simulink model "check_serial_new_arduino_basic"  (R2021a)
settings: Solver=FixedStepDiscrete  StartTime=0.0  StopTime=inf  FixedStep=time_step  RelTol=1e-3
model workspace (MAT data in the model file):
  time_step = 0.01
undefined symbols (not defined in the file): Serial_Port, Standard_Devices
libraries: sldrtlib x2
settings Model: Creator=Rahul Subramanian  LastModifiedBy=Rahul Subramanian
settings SolverCC: AlgebraicLoopSolver=TrustRegion
settings DebuggingCC: SFMachineParentedDataDiag=warning
settings RTWCC: Description=Simulink Desktop Real-Time  SystemTargetFile=sldrt.tlc  TemplateMakefile=sldrt.tmf  RTWCompilerOptimization=on
settings CodeAppCC: MaxIdLength=95
settings SimulinkDesktopRealTimeCC: TargetPreCompLibLocation=C:\Program Files\MATLAB\R2021a\toolbox\sldrt\lib\win64

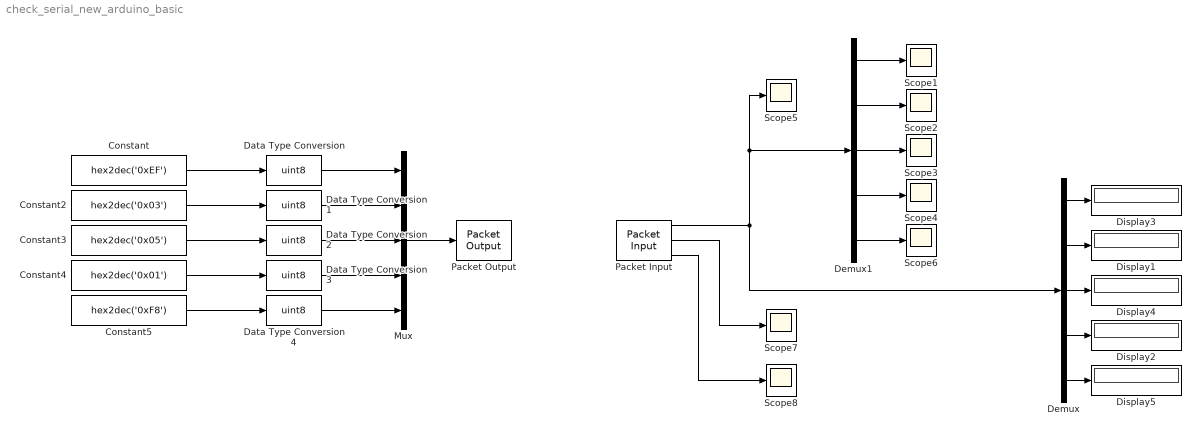
== system check_serial_new_arduino_basic ==
  Constant : Constant  Value=hex2dec('0xEF')
  Constant2 : Constant  Value=hex2dec('0x03')
  Constant3 : Constant  Value=hex2dec('0x05')
  Constant4 : Constant  Value=hex2dec('0x01')
  Constant5 : Constant  Value=hex2dec('0xF8')
  Data Type Conversion{,1..4} (5 alike) : DataTypeConversion  OutDataTypeStr=uint8
  Demux : Demux  Outputs=5
  Demux1 : Demux  Outputs=5
  Display{1..5} (5 alike) : Display
      settings: Format=hex (Stored Integer)
  Mux : Mux  Inputs=5
  Packet Input : sldrtlib/Packet Input  SampleTime=0.1  MaxMissedTicks=10  ShowMissedTicks=off  YieldWhenWaiting=off  DrvName=Standard_Devices/Serial_Port  DrvAddress=5  DrvOptions=[115200 8 0 0 0 0 0 0]  PacketSize=5  DataTypes='5*uint8'  ShowReady=on  ShowError=on  PacketID=1  ByteOrder=1  ShowTimestamp=off
      settings: AttributesFormatString=Serial Port [5]
  Packet Output : sldrtlib/Packet Output  SampleTime=0.1  MaxMissedTicks=10  ShowMissedTicks=off  YieldWhenWaiting=off  DrvName=Standard_Devices/Serial_Port  DrvAddress=5  DrvOptions=[115200 8 0 0 0 0 0 0]  PacketSize=5  DataTypes='5*uint8'  ShowReady=off  ShowError=off  PacketID=1  ByteOrder=1  InitialValue=[]  FinalValue=[]
      settings: AttributesFormatString=Serial Port [5]
  Scope{1..8} (8 alike) : Scope
  wires:
  Constant/1 -> Data Type Conversion/1
  Constant2/1 -> Data Type Conversion1/1
  Constant3/1 -> Data Type Conversion2/1
  Constant4/1 -> Data Type Conversion3/1
  Constant5/1 -> Data Type Conversion4/1
  Data Type Conversion/1 -> Mux/1
  Data Type Conversion1/1 -> Mux/2
  Data Type Conversion2/1 -> Mux/3
  Data Type Conversion3/1 -> Mux/4
  Data Type Conversion4/1 -> Mux/5
  Packet Input/1 -> Demux/1, Demux1/1, Scope5/1
  Packet Input/2 -> Scope7/1
  Packet Input/3 -> Scope8/1
  Demux/2 -> Display1/1
  Demux/1 -> Display3/1
  Demux/3 -> Display4/1
  Demux/4 -> Display2/1
  Demux/5 -> Display5/1
  Mux/1 -> Packet Output/1
  Demux1/1 -> Scope1/1
  Demux1/2 -> Scope2/1
  Demux1/3 -> Scope3/1
  Demux1/4 -> Scope4/1
  Demux1/5 -> Scope6/1
